simulink model "Demo_SecOrder_TVP"  (R2014b)
settings: Solver=ode4  StartTime=0.0  StopTime=tend  FixedStep=Ts  RelTol=1e-3
values from neighbouring files (symbols this model uses):
  Ts = 0.1    [contsid_EIV.m]    (also in contsid_Hammerstein2.m = 0.5; contsid_LPV.m = 0.005; contsid_MIMO2.m; contsid_advantage21.m = k*(0.1-0.01)+ 0.01)
undefined symbols (not defined in the file or in its folder): varv
settings Model: Creator=Mathieu  LastModifiedBy=arturo
settings DataIOCC: SignalLoggingSaveFormat=ModelDataLogs
settings OptimizationCC: ExpressionDepthLimit=2147483647
settings DebuggingCC: UnderspecifiedInitializationDetection=Classic  MergeDetectMultiDrivingBlocksExec=none  FcnCallInpInsideContextMsg=UseLocalSettings  StateNameClashWarn=warning
settings GRTTargetCC: CombineOutputUpdateFcns=off  GRTInterface=on

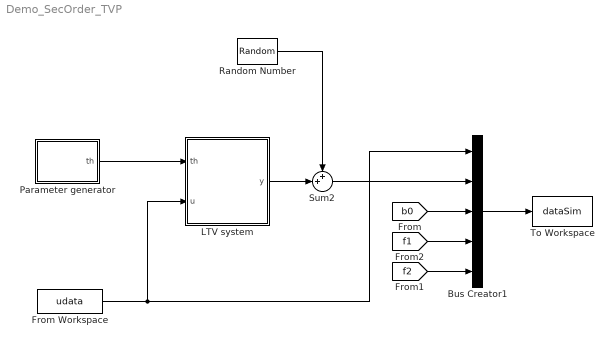
== system Demo_SecOrder_TVP ==
  Bus Creator1 : BusCreator  Inputs=5
  From Workspace : FromWorkspace  VariableName=udata  SampleTime=Ts
  LTV system : Subsystem
  Parameter generator : Subsystem
  Random Number : RandomNumber  Variance=varv  SampleTime=0
  Sum2 : Sum  Inputs=++|
  To Workspace : ToWorkspace  VariableName=dataSim  SampleTime=Ts
  wires:
  Bus Creator1/1 -> To Workspace/1
  From Workspace/1 -> Bus Creator1/1, LTV system/2(u)
  [b0] -> Bus Creator1/3
  [f2] -> Bus Creator1/5
  [f1] -> Bus Creator1/4
  LTV system/1(y) -> Sum2/2
  Sum2/1 -> Bus Creator1/2
  Random Number/1 -> Sum2/1
  Parameter generator/1(th) -> LTV system/1(th)

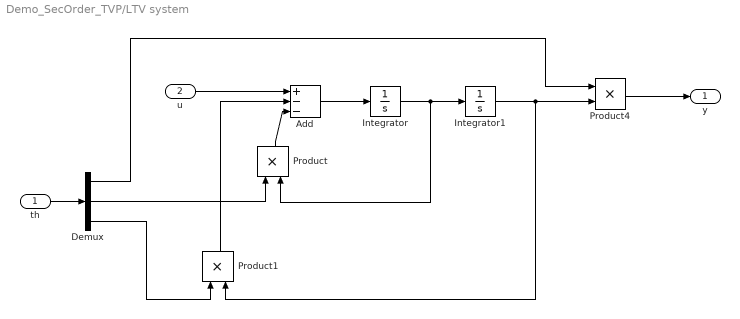
== system Demo_SecOrder_TVP/LTV system ==
  th : Inport
  u : Inport  Port=2
  Add : Sum  Inputs=+--
  Demux : Demux  Outputs=3
  Integrator : Integrator
  Integrator1 : Integrator
  Product : Product
  Product1 : Product
  Product4 : Product  RndMeth=Zero
  y : Outport
  wires:
  Product1/1 -> Add/2
  Add/1 -> Integrator/1
  Product/1 -> Add/3
  Integrator1/1 -> Product4/2, Product1/2
  Integrator/1 -> Integrator1/1, Product/2
  Demux/1 -> Product4/1
  u/1 -> Add/1
  Product4/1 -> y/1
  Demux/2 -> Product/1
  Demux/3 -> Product1/1
  th/1 -> Demux/1

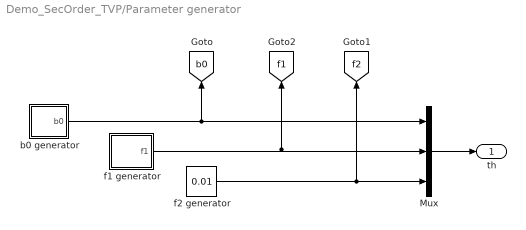
== system Demo_SecOrder_TVP/Parameter generator ==
  Mux : Mux  Inputs=3
  b0 generator : Subsystem
  f1 generator : Subsystem
  f2 generator : Constant  Value=0.01
  th : Outport
  tag scope: b0=global, f1=global, f2=global
  wires:
  f2 generator/1 -> Mux/3, [f2]
  b0 generator/1(b0) -> Mux/1, [b0]
  f1 generator/1(f1) -> Mux/2, [f1]
  Mux/1 -> th/1

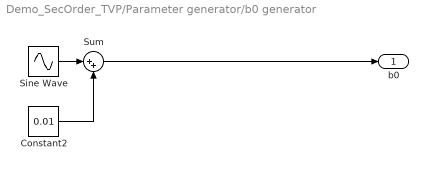
== system Demo_SecOrder_TVP/Parameter generator/b0 generator ==
  Constant2 : Constant  Value=0.01
  Sine Wave : Sin  Amplitude=0.008  Frequency=2*pi/(1e4/3)  SampleTime=0
  Sum : Sum  Inputs=|++
  b0 : Outport
  wires:
  Sine Wave/1 -> Sum/1
  Sum/1 -> b0/1
  Constant2/1 -> Sum/2

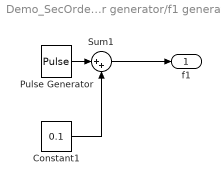
== system Demo_SecOrder_TVP/Parameter generator/f1 generator ==
  Constant1 : Constant  Value=0.1
  Pulse Generator : DiscretePulseGenerator  PulseType=Time based  Amplitude=0.09  Period=12000  PulseWidth=75
  Sum1 : Sum  Inputs=|++
  f1 : Outport
  wires:
  Pulse Generator/1 -> Sum1/1
  Sum1/1 -> f1/1
  Constant1/1 -> Sum1/2
